simulink library "mylib"  (R2023a)
settings: Solver=VariableStepAuto  StartTime=0.0  StopTime=10.0  RelTol=1e-3
libraries: fl_lib x16, nesl_utility x10, simulink x4, ee_lib x1, $bdroot x1
settings Model: Creator=Erlend  LastModifiedBy=tormod
settings DebuggingCC: UnconnectedInputMsg=warning  UnconnectedOutputMsg=warning  UnconnectedLineMsg=warning
settings ModelReferenceCC: EnableRefExpFcnMdlSchedulingChecks=on
settings RTWCC: DLArmComputeVersion=19.05

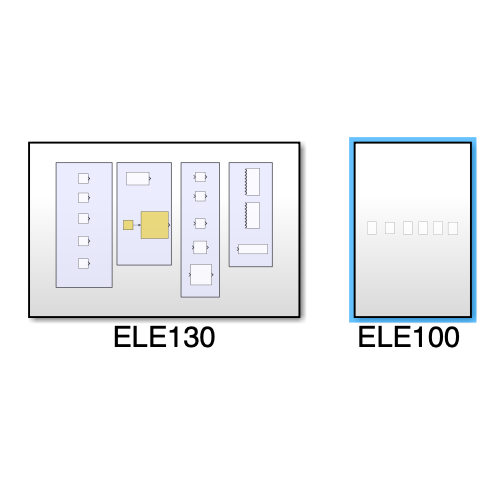
[thumbnail: Simulink's stored preview of the top-level diagram]
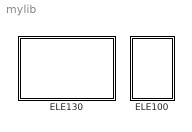
== system mylib ==
  "ELE100 " : Subsystem
  ELE130 : Subsystem

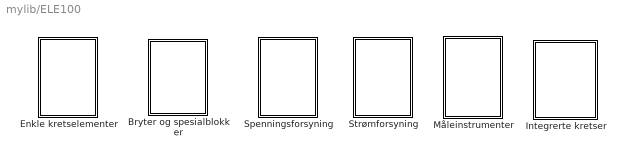
== system mylib/ELE100  ==
  Bryter og spesialblokker : Subsystem
  Enkle kretselementer : Subsystem
  Integrerte kretser : Subsystem
  Måleinstrumenter : Subsystem
  Spenningsforsyning : Subsystem
  Strømforsyning : Subsystem

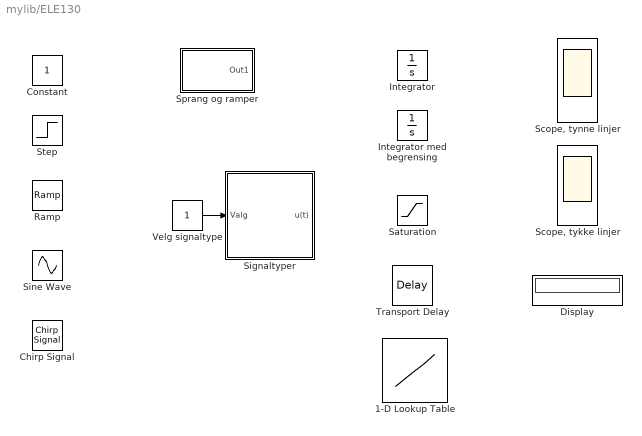
== system mylib/ELE130 ==
  1-D Lookup Table : Lookup_n-D  NumberOfTableDimensions=1  BreakpointsForDimension1=[0:0.1:1]  Table=rand(1,11)  InternalRulePriority=Speed  RndMeth=Simplest
      settings: AttributesFormatString=|
      | INN = %<BreakpointsForDimension1>
      | UT = %<Table>
  Chirp Signal : simulink/Sources/Chirp Signal  f1=0.1  T=100  f2=1
      settings: AttributesFormatString=|
      | u(t) = sin(2 pi f(t) t)
      | f(t) = %<f1> + (%<f2>-%<f1>)/%<T>*t   [Hz]
  Constant : Constant
  Display : Display
  Integrator : Integrator
      settings: AttributesFormatString=IC = %<InitialCondition>
  Integrator med begrensing : Integrator  LimitOutput=on
      settings: AttributesFormatString=|
      | IC = %<InitialCondition>
      | Max = %<UpperSaturationLimit>
      | Min = %<LowerSaturationLimit>
  Ramp : simulink/Sources/Ramp  slope=0.03  start=5  InitialOutput=2
      settings: AttributesFormatString="u(t) = %<InitialOutput>  + %<slope> (t - %<start>)"
  Saturation : Saturate
      settings: AttributesFormatString=|
      | Max = %<UpperLimit>
      | Min = %<LowerLimit>
  "Scope, tykke linjer" : Scope  NumInputPorts=8
  "Scope, tynne linjer" : Scope  NumInputPorts=8
  Signaltyper : Subsystem
      mask Display:
      | disp(['Signaltyper:      \n',...
      | ' 1: konstant       \n',...
      | ' 2: sprang         \n',...
      | ' 3: rampe          \n',...
      | ' 4: egendefinert\n',...
      | ' 5: sinus            \n',...
      | ' 6: chirp            '])
  Sine Wave : Sin  SampleTime=0
      settings: AttributesFormatString=u(t) = %<Amplitude> sin(%<Frequency>t + %<Phase>) + %<Bias>
  Sprang og ramper : Subsystem  mask{tidspunkt=[0 1 2 3 4 5], utgangsverdi=[0 0 1 -1 0 0], valg=Trappetrinn}
      mask prompts: tidspunkt "Tidspunkter (vektorform)"; utgangsverdi "Utgangsverdier (vektorform)"; valg "Interpolasjonsmetode"
      settings: AttributesFormatString=|
      | t = %<tidspunkt>
      | u = %<utgangsverdi>
      mask TypeOptions valg: Trappetrinn | Linear
      mask Display:
      | if valg==1
      |     [tt,yy]=stairs(tidspunkt,utgangsverdi);
      |     tt=[tt;tt(end)*1.2];
      |     yy=[yy;yy(end)];
      |     plot(tt,yy)
      | elseif valg==2
      |     plot(tidspunkt,utgangsverdi);
      | end
  Step : Step  SampleTime=0
      settings: AttributesFormatString=|
      | u(t) = %<Before> for t < %<Time>s
      |       = %<After> for t > %<Time>s
  Transport Delay : TransportDelay  DelayTime=2
      settings: AttributesFormatString=delay = %<DelayTime>s
  Velg signaltype : Constant
  wires:
  Velg signaltype/1 -> Signaltyper/1(Valg)

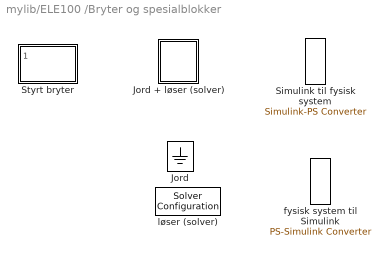
== system mylib/ELE100 /Bryter og spesialblokker ==
  Jord : fl_lib/Electrical/Electrical Elements/Electrical Reference
  Jord + løser (solver) : Subsystem
      settings: PortSchema="{\"entries\":[{\"content\":{\"sides\":[{\"content\":{\"connectorIds\":[]},\"type\":\"ConnectorPlacement.EquallySpacedRectSide\",\"uuid\":\"d6eeaf75-7a7b-4c6b-8fcc-970490e66e70\"},{\"content\":{\"connectorIds\":[],\"side\":\"RIGHT\"},\"type\":\"ConnectorPlacement.EquallySpacedRectSide\",\"uuid\":\"40329f91-e021-44b2-b457-2c61881d9cd9\"},{\"content\":{\"connectorIds\":[\"LConn1\"],\"side\":\"TOP\"},\"type\":\"ConnectorPlacement.EquallySpacedRectSide\",\"uuid\":\"55ef3106-c83b-48b0-b585-fed4149e4501\"}]},\"type\":\"ConnectorPlacement.EquallySpacedConnector\",\"uuid\":\"04a40fb0-bc21-4b12-952a-4fb2fac27a5d\"}],\"packageUris\":[\"http://schema.mathworks.com/mf0/Connector/R2020b\"],\"version\":\"1.0\"}"
      mask Display:
      | plot([-2 2], [1.5 1.5])
      | plot([-1.5 1.5], [0.75 0.75])
      | plot([-1 1], [0 0])
      | plot([-0.5 0.5], [-0.75 -0.75])
      | plot([0 0], [-1.5 -1.5])
      | plot([0 0], [3 1.5])
  Simulink til fysisk system : nesl_utility/Simulink-PS Converter  PhysicalDomain=network_engine_domain  SubClassName=ps_input  LeftPortType=input  RightPortType=output  PseudoPeriodic=off  Frequencies=[]  NoiseDistribution=none  NoiseParameters=[]  Unit=1  AffineConversion=off  FilteringAndDerivatives=provide  SimscapeFilterOrder=1  InputFilterTimeConstant=0.001  UdotUserProvided=0
  Styrt bryter : Subsystem
      mask Display:
      | plot([4 4],[0 3])
      | plot([0 4],[3 3])
      | plot([0,3],[1 1])
      | plot([3,5],[-1 1])
      | plot([5,7],[1 1])
      | text(4.5,2,'0/1')
      | plot([0 0],[4 4])
      | plot([0 0],[-1.5 -1.5])
  "fysisk system til Simulink " : nesl_utility/PS-Simulink Converter  PhysicalDomain=network_engine_domain  SubClassName=ps_output  LeftPortType=input  RightPortType=output  PseudoPeriodic=off  Frequencies=[]  VectorFormat=1-D array  Unit=inherit  AffineConversion=off
  "løser (solver) " : nesl_utility/Solver Configuration  PhysicalDomain=network_engine_domain  SubClassName=solver  LeftPortType=input  RightPortType=generic  Tones=[]  Harmonics=[]  SimulateNoise=off  Profile=off  UseLocalSampling=off  EnableSwitchedLinearOptims=on  FrequencyDomain=off  UseCCode=off  RelTol=0.001  AbsTol=1e-06  MinStep=1e-09  ToWorkspace=off  RevertToSquareIcSolve=off  NumHomotopyIterations=100  PhasorMode=off  PhasorModeNumHarmonics=1  ConsistencySolver=NEWTON_FTOL  IndexReductionMethod=DerivativeReplacement  DoDC=off  ResidualTolerance=1e-09  ConsistencyTolSource=GLOBAL  ConsistencyAbsTol=0.001  ConsistencyRelTol=0.001  ConsistencyTolFactor=0.001  UseLocalSolver=off  LocalSolverChoice=NE_BACKWARD_EULER_ADVANCER  ResolveIndetEquations=on  FunctionEvalNumThread=1  LocalSolverSampleTime=0.001  DoFixedCost=off  MaxNonlinIter=3  MaxModeIter=2  ComputeImpulses=off  ImpulseIterations=2  LinearAlgebra=Sparse  LinearAlgebraNumThread=0  EquationFormulation=NE_TIME_EF  DelaysMemoryBudget=1024  AutomaticFiltering=on  FilteringTimeConstant=0.001  PartitionStorageMethod=AS_NEEDED  PartitionMemoryBudget=1024  PartitionMethod=FAST

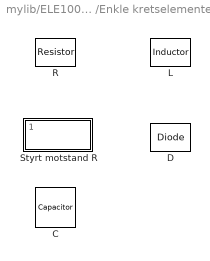
== system mylib/ELE100 /Enkle kretselementer ==
  C : fl_lib/Electrical/Electrical Elements/Capacitor  c=1 uF  r=1e-6 Ohm  g=0 1/Ohm  i_specify=off  i_priority=None  i=0 A  i_nominal_specify=off  i_nominal_unit=A  i_nominal_value=1  v_specify=off  v_priority=None  v=0 V  v_nominal_specify=off  v_nominal_unit=V  v_nominal_value=1  vc_specify=off  vc_priority=High  vc=0 V  vc_nominal_specify=off  vc_nominal_unit=V  vc_nominal_value=1
      settings: AttributesFormatString=%<c> %<c_unit>
  D : fl_lib/Electrical/Electrical Elements/Diode  Vf=0.6 V  Ron=0.3 Ohm  Goff=1e-8 1/Ohm  i_specify=off  i_priority=None  i=0 A  i_nominal_specify=off  i_nominal_unit=A  i_nominal_value=1  v_specify=off  v_priority=None  v=0 V  v_nominal_specify=off  v_nominal_unit=V  v_nominal_value=1
      settings: AttributesFormatString=|
      | Vf=%<Vf> %<Vf_unit>
      | R_on=%<Ron> %<Ron_unit>
  L : fl_lib/Electrical/Electrical Elements/Inductor  l=100 nH  r=0 Ohm  g=1e-9 1/Ohm  i_specify=off  i_priority=None  i=0 A  i_nominal_specify=off  i_nominal_unit=A  i_nominal_value=1  v_specify=off  v_priority=None  v=0 V  v_nominal_specify=off  v_nominal_unit=V  v_nominal_value=1  i_L_specify=off  i_L_priority=High  i_L=0 A  i_L_nominal_specify=off  i_L_nominal_unit=A  i_L_nominal_value=1
      settings: AttributesFormatString=%<l> %<l_unit>
  R : fl_lib/Electrical/Electrical Elements/Resistor  R=50 Ohm  i_specify=off  i_priority=None  i=0 A  i_nominal_specify=off  i_nominal_unit=A  i_nominal_value=1  v_specify=off  v_priority=None  v=0 V  v_nominal_specify=off  v_nominal_unit=V  v_nominal_value=1
      settings: AttributesFormatString=%<R> %<R_unit>
  Styrt motstand R : Subsystem
      mask Display:
      | plot([0 1 1 2 2 3 3 4 4 5 5 6 6 7 7],[-1 1 1 -1 -1 1 1 -1 -1 1 1 -1 -1 1 1])
      | plot([4 4],[0 3])
      | plot([0 4],[3 3])
      | plot([3.5 4],[0.7 0])
      | plot([4 4.5],[0 0.7])
      | plot([0 0],[4 4])
      | plot([0 0],[-1.5 -1.5])

== system mylib/ELE100 /Integrerte kretser ==
  Operasjonsforsterkar : ee_lib/Integrated Circuits/Band-Limited Op-Amp  A=100000  Rin=1e12 Ohm  Rout=20 Ohm  Vmin=-5 V  Vmax=5 V  Vdotmax=1e6 V/s  f=10 Hz  V0=0 V
      settings: AttributesFormatString=|
      | Forsterking A_o = %<A>
      | Bandbreidde f_o = %<f> %<f_unit>

== system mylib/ELE100 /Måleinstrumenter ==
  i_navn : Subsystem
      mask Display:
      | t=0:0.01:2*pi;
      | y=sin(t);
      | x=cos(t);
      | plot(x,y)
      | text(-0.2,-0.1,'A')
      | plot(2,2)
      | plot(-2.1,-2)
      | plot([-2,-1],[0,0])
      | plot([1,1.5],[0,0])
      | plot([1.5,1.5],[0,-0.8])
      | plot([1.5,2.3],[-0.8,-0.8])
      | text(-1.8,0.6,'+')
      | text(1.5,-0.7,'_')
  v_navn : Subsystem
      mask Display:
      | t=0:0.01:2*pi;
      | y=sin(t);
      | x=cos(t);
      | plot(x,y)
      | plot([0 0],[-1.5 -1])
      | plot([0 0],[1 1.5])
      | text(-0.2,-0.1,'V')
      | plot(1.5,2)
      | plot(-2.3,-2)
      | plot([-2.4,0],[1.5,1.5])
      | plot([-2.4,0],[-1.5,-1.5])
      | text(-1.9,0.8,'+')
      | text(-1.9,-0.4,'_')

== system mylib/ELE100 /Spenningsforsyning ==
  Styrt spenning v_S : Subsystem
      mask Display:
      | t=0:0.01:2*pi;
      | y=sin(t);
      | x=cos(t);
      | plot(x,y)
      | plot([-1.5 1.5],[1.5 -1.5])
      | plot([1.3 1.5],[-1 -1.5])
      | plot([1.05 1.5],[-1.25 -1.5])
      | plot([-2 -1],[0 0])
      | plot([1 2],[0 0])
      | text(0.5,0,'+')
      | text(-0.5,0,'-')
  V_S : fl_lib/Electrical/Electrical Sources/DC Voltage Source  v0=1 V
      settings: AttributesFormatString=%<v0> %<v0_unit> DC
  V_S_ac : fl_lib/Electrical/Electrical Sources/AC Voltage Source  amp=1 V  shift=0 deg  frequency=10 Hz  omega=0 rad/s
      settings: AttributesFormatString=|
      | %<amp> %<amp_unit> AC
      | %<frequency> %<frequency_unit>

== system mylib/ELE100 /Strømforsyning ==
  I_S : fl_lib/Electrical/Electrical Sources/DC Current Source  i0=1 A
      settings: AttributesFormatString=%<i0> %<i0_unit> DC  InternalSimscapePortConfiguration="{\"Bottom\":[],\"Left\":[{\"id\":\"p\",\"label\":\"\",\"type\":\"foundation.electrical.electrical\"}],\"Right\":[{\"id\":\"n\",\"label\":\"\",\"type\":\"foundation.electrical.electrical\"}],\"Top\":[]}"
  I_S_ac : fl_lib/Electrical/Electrical Sources/AC Current Source  amp=1 A  shift=0 deg  frequency=60 Hz  omega=0 rad/s
      settings: InternalSimscapePortConfiguration="{\"Bottom\":[],\"Left\":[{\"id\":\"p\",\"label\":\"\",\"type\":\"foundation.electrical.electrical\"}],\"Right\":[{\"id\":\"n\",\"label\":\"\",\"type\":\"foundation.electrical.electrical\"}],\"Top\":[]}"
      settings: AttributesFormatString=|
      | %<amp> %<amp_unit> AC
      | %<frequency> %<frequency_unit>
  Styrt strøm i_S : Subsystem
      mask Display:
      | t=0:0.01:2*pi;
      | y=sin(t);
      | x=cos(t);
      | plot(x,y)
      | plot([1.5 -1.5],[-1.5 1.5])
      | plot([1.3 1.5],[-1 -1.5])
      | plot([1.05 1.5],[-1.25 -1.5])
      | plot([-2 -1],[0 0])
      | plot([1 2],[0 0])
      | plot([-0.5 0.5],[0 0])
      | plot([0.3 0.5],[-0.15 0])
      | plot([0.3 0.5],[0.15 0])

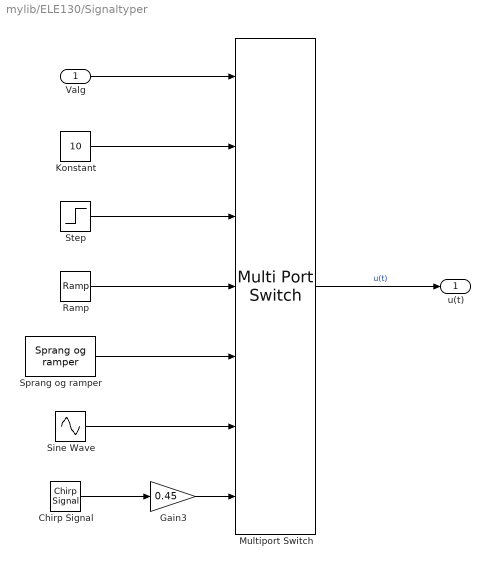
== system mylib/ELE130/Signaltyper ==
  Valg : Inport
  Chirp Signal : simulink/Sources/Chirp Signal  f1=0.1  T=100  f2=1
      settings: AttributesFormatString=|
      | u(t) = sin(2 pi f(t) t)
      | f(t) = %<f1> + (%<f2> - %<f1>)/%<T>s*t [Hz]
  Gain3 : Gain  Gain=0.45
      settings: AttributesFormatString=ampl = %<Gain>
  Konstant : Constant  Value=10
  Multiport Switch : MultiPortSwitch  Inputs=6  SaturateOnIntegerOverflow=off  InputSameDT=off
  Ramp : simulink/Sources/Ramp  slope=0.03  start=5  InitialOutput=2
      settings: AttributesFormatString="u(t) = %<InitialOutput>  + %<slope> (t - %<start>)"
  Sine Wave : Sin  SampleTime=0
      settings: AttributesFormatString=u(t) = %<Amplitude> sin(%<Frequency>t + %<Phase>) + %<Bias>
  Sprang og ramper : $bdroot/ELE130/Sprang og ramper  tidspunkt=[0 1 2 3 4 5]  utgangsverdi=[0 0 1 -1 0 0]  valg=Trappetrinn
      settings: AttributesFormatString=|
      | t = %<tidspunkt>
      | u = %<utgangsverdi>
  Step : Step  SampleTime=0
      settings: AttributesFormatString=|
      | u(t) = %<Before> for t < %<Time>s
      |       = %<After> for t > %<Time>s
  u(t) : Outport
  wires:
  Multiport Switch/1 -> u(t)/1  "u(t)"
  Valg/1 -> Multiport Switch/1
  Chirp Signal/1 -> Gain3/1
  Konstant/1 -> Multiport Switch/2
  Sine Wave/1 -> Multiport Switch/6
  Gain3/1 -> Multiport Switch/7
  Sprang og ramper/1 -> Multiport Switch/5
  Ramp/1 -> Multiport Switch/4
  Step/1 -> Multiport Switch/3

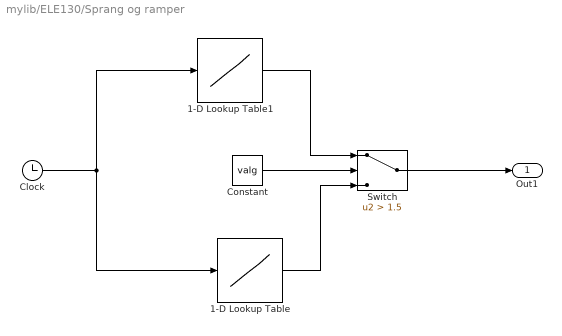
== system mylib/ELE130/Sprang og ramper ==
  1-D Lookup Table : Lookup_n-D  NumberOfTableDimensions=1  BreakpointsForDimension1=tidspunkt  Table=utgangsverdi  InterpMethod=Flat  RndMeth=Simplest
      settings: AttributesFormatString=%<InterpMethod>
  1-D Lookup Table1 : Lookup_n-D  NumberOfTableDimensions=1  BreakpointsForDimension1=tidspunkt  Table=utgangsverdi  RndMeth=Simplest
      settings: AttributesFormatString=%<InterpMethod>
  Clock : Clock
  Constant : Constant  Value=valg
  Switch : Switch  Criteria=u2 > Threshold  Threshold=1.5  SaturateOnIntegerOverflow=off  InputSameDT=off
  Out1 : Outport  VectorParamsAs1DForOutWhenUnconnected=off
  wires:
  Clock/1 -> 1-D Lookup Table1/1, 1-D Lookup Table/1
  1-D Lookup Table/1 -> Switch/3
  1-D Lookup Table1/1 -> Switch/1
  Switch/1 -> Out1/1
  Constant/1 -> Switch/2

== system mylib/ELE100 /Bryter og spesialblokker/Jord + løser (solver) ==
  Electrical Reference : fl_lib/Electrical/Electrical Elements/Electrical Reference
  Solver Configuration : nesl_utility/Solver Configuration  PhysicalDomain=network_engine_domain  SubClassName=solver  LeftPortType=input  RightPortType=generic  Tones=[]  Harmonics=[]  SimulateNoise=off  Profile=off  UseLocalSampling=off  EnableSwitchedLinearOptims=on  FrequencyDomain=off  UseCCode=off  RelTol=0.001  AbsTol=1e-06  MinStep=1e-09  ToWorkspace=off  RevertToSquareIcSolve=off  NumHomotopyIterations=100  PhasorMode=off  PhasorModeNumHarmonics=1  ConsistencySolver=NEWTON_FTOL  IndexReductionMethod=DerivativeReplacement  DoDC=off  ResidualTolerance=1e-09  ConsistencyTolSource=GLOBAL  ConsistencyAbsTol=0.001  ConsistencyRelTol=0.001  ConsistencyTolFactor=0.001  UseLocalSolver=off  LocalSolverChoice=NE_BACKWARD_EULER_ADVANCER  ResolveIndetEquations=on  FunctionEvalNumThread=1  LocalSolverSampleTime=0.001  DoFixedCost=off  MaxNonlinIter=3  MaxModeIter=2  ComputeImpulses=off  ImpulseIterations=2  LinearAlgebra=Sparse  LinearAlgebraNumThread=0  EquationFormulation=NE_TIME_EF  DelaysMemoryBudget=1024  AutomaticFiltering=on  FilteringTimeConstant=0.001  PartitionStorageMethod=AS_NEEDED  PartitionMemoryBudget=1024  PartitionMethod=FAST
  Connection Port : PMIOPort  Side=Left
  connections:
  Electrical Reference/LConn1 -- Solver Configuration/RConn1 -- Connection Port/RConn1

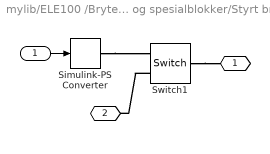
== system mylib/ELE100 /Bryter og spesialblokker/Styrt bryter ==
  "   " : Inport
  Simulink-PS Converter : nesl_utility/Simulink-PS Converter  PhysicalDomain=network_engine_domain  SubClassName=ps_input  LeftPortType=input  RightPortType=output  PseudoPeriodic=off  Frequencies=[]  NoiseDistribution=none  NoiseParameters=[]  Unit=1  AffineConversion=off  FilteringAndDerivatives=zero  SimscapeFilterOrder=1  InputFilterTimeConstant=0.001  UdotUserProvided=1
  Switch1 : fl_lib/Electrical/Electrical Elements/Switch  R_closed=0.01 Ohm  G_open=1e-8 1/Ohm  Threshold=0  i_specify=off  i_priority=None  i=0 A  i_nominal_specify=off  i_nominal_unit=A  i_nominal_value=1  v_specify=off  v_priority=None  v=0 V  v_nominal_specify=off  v_nominal_unit=V  v_nominal_value=1
  "  " : PMIOPort  Side=Left
  " " : PMIOPort  Port=2  Side=Right
  wires:
  "   "/1 -> Simulink-PS Converter/1
  connections:
  Simulink-PS Converter/RConn1 -- Switch1/RConn1
  Switch1/RConn2 -- " "/RConn1
  Switch1/LConn1 -- "  "/RConn1

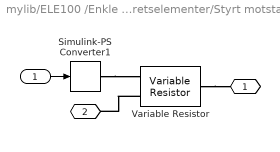
== system mylib/ELE100 /Enkle kretselementer/Styrt motstand R ==
  "      " : Inport
  Simulink-PS Converter1 : nesl_utility/Simulink-PS Converter  PhysicalDomain=network_engine_domain  SubClassName=ps_input  LeftPortType=input  RightPortType=output  PseudoPeriodic=off  Frequencies=[]  NoiseDistribution=none  NoiseParameters=[]  Unit=1  AffineConversion=off  FilteringAndDerivatives=zero  SimscapeFilterOrder=1  InputFilterTimeConstant=0.001  UdotUserProvided=1
  Variable Resistor : fl_lib/Electrical/Electrical Elements/Variable Resistor  Rmin=0 Ohm  i_specify=off  i_priority=None  i=0 A  i_nominal_specify=off  i_nominal_unit=A  i_nominal_value=1  v_specify=off  v_priority=None  v=0 V  v_nominal_specify=off  v_nominal_unit=V  v_nominal_value=1
  "     " : PMIOPort  Side=Right
  "  " : PMIOPort  Port=2  Side=Left
  wires:
  "      "/1 -> Simulink-PS Converter1/1
  connections:
  Simulink-PS Converter1/RConn1 -- Variable Resistor/LConn1
  Variable Resistor/LConn2 -- "  "/RConn1
  Variable Resistor/RConn1 -- "     "/RConn1

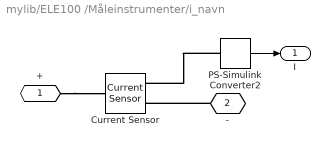
== system mylib/ELE100 /Måleinstrumenter/i_navn ==
  Current Sensor : fl_lib/Electrical/Electrical Sensors/Current Sensor
  PS-Simulink Converter2 : nesl_utility/PS-Simulink Converter  PhysicalDomain=network_engine_domain  SubClassName=ps_output  LeftPortType=input  RightPortType=output  PseudoPeriodic=off  Frequencies=[]  VectorFormat=1-D array  Unit=1  AffineConversion=off
  + : PMIOPort  Side=Left
  - : PMIOPort  Port=2  Side=Right
  " I" : Outport  VectorParamsAs1DForOutWhenUnconnected=off
  wires:
  PS-Simulink Converter2/1 -> " I"/1
  connections:
  PS-Simulink Converter2/LConn1 -- Current Sensor/RConn1
  +/RConn1 -- Current Sensor/LConn1
  -/RConn1 -- Current Sensor/RConn2

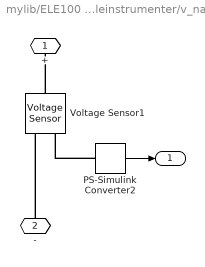
== system mylib/ELE100 /Måleinstrumenter/v_navn ==
  PS-Simulink Converter2 : nesl_utility/PS-Simulink Converter  PhysicalDomain=network_engine_domain  SubClassName=ps_output  LeftPortType=input  RightPortType=output  PseudoPeriodic=off  Frequencies=[]  VectorFormat=1-D array  Unit=1  AffineConversion=off
  Voltage Sensor1 : fl_lib/Electrical/Electrical Sensors/Voltage Sensor
  + : PMIOPort  Side=Left
  - : PMIOPort  Port=2  Side=Left
  " " : Outport  VectorParamsAs1DForOutWhenUnconnected=off
  wires:
  PS-Simulink Converter2/1 -> " "/1
  connections:
  PS-Simulink Converter2/LConn1 -- Voltage Sensor1/RConn1
  Voltage Sensor1/LConn1 -- +/RConn1
  -/RConn1 -- Voltage Sensor1/RConn2

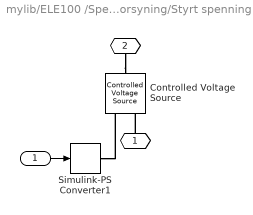
== system mylib/ELE100 /Spenningsforsyning/Styrt spenning v_S ==
  "  " : Inport
  Controlled Voltage Source : fl_lib/Electrical/Electrical Sources/Controlled Voltage Source
  Simulink-PS Converter1 : nesl_utility/Simulink-PS Converter  PhysicalDomain=network_engine_domain  SubClassName=ps_input  LeftPortType=input  RightPortType=output  PseudoPeriodic=off  Frequencies=[]  NoiseDistribution=none  NoiseParameters=[]  Unit=1  AffineConversion=off  FilteringAndDerivatives=zero  SimscapeFilterOrder=1  InputFilterTimeConstant=0.001  UdotUserProvided=1
  " " : PMIOPort  Side=Left
  "   " : PMIOPort  Port=2  Side=Right
  wires:
  "  "/1 -> Simulink-PS Converter1/1
  connections:
  Simulink-PS Converter1/RConn1 -- Controlled Voltage Source/RConn1
  "   "/RConn1 -- Controlled Voltage Source/LConn1
  " "/RConn1 -- Controlled Voltage Source/RConn2

== system mylib/ELE100 /Strømforsyning/Styrt strøm i_S ==
  "  " : Inport
  Controlled Current Source : fl_lib/Electrical/Electrical Sources/Controlled Current Source
  Simulink-PS Converter1 : nesl_utility/Simulink-PS Converter  PhysicalDomain=network_engine_domain  SubClassName=ps_input  LeftPortType=input  RightPortType=output  PseudoPeriodic=off  Frequencies=[]  NoiseDistribution=none  NoiseParameters=[]  Unit=1  AffineConversion=off  FilteringAndDerivatives=zero  SimscapeFilterOrder=1  InputFilterTimeConstant=0.001  UdotUserProvided=1
  " " : PMIOPort  Side=Left
  "   " : PMIOPort  Port=2  Side=Right
  wires:
  "  "/1 -> Simulink-PS Converter1/1
  connections:
  Controlled Current Source/RConn1 -- Simulink-PS Converter1/RConn1
  "   "/RConn1 -- Controlled Current Source/LConn1
  " "/RConn1 -- Controlled Current Source/RConn2
